simulink model "SS_F16_Block"  (Simulink 10.0)
settings: Solver=ode5  StartTime=0.0  StopTime=50  FixedStep=0.001  RelTol=1e-3  EnableMultiTasking=on
values from neighbouring files (symbols this model uses):
  A = A_lo    [augumentedF16.m]    (also in my_runLINF16sim.m; runLINF16sim.m)
  B = B_lo    [augumentedF16.m]    (also in my_runLINF16sim.m; runLINF16sim.m)
  C = C_lo    [augumentedF16.m]    (also in my_runLINF16sim.m; runLINF16sim.m)
  D = D_lo    [augumentedF16.m]    (also in my_runLINF16sim.m; runLINF16sim.m)
  DisAil_1 = AileronDis    (= 0)    [augumentedF16.m]    (also in my_runF16Sim.m; my_runLINF16sim.m; runF16Sim.m; runLINF16sim.m)
  DisAil_2 = -2*AileronDis    (= 0)    [augumentedF16.m]    (also in my_runF16Sim.m; my_runLINF16sim.m; runF16Sim.m; runLINF16sim.m)
  DisAil_3 = AileronDis    (= 0)    [augumentedF16.m]    (also in my_runF16Sim.m; my_runLINF16sim.m; runF16Sim.m; runLINF16sim.m)
  DisEle_1 = ElevatorDis    (= 0)    [augumentedF16.m]    (also in my_runF16Sim.m; my_runLINF16sim.m; runF16Sim.m; runLINF16sim.m)
  DisEle_2 = -2*ElevatorDis    (= 0)    [augumentedF16.m]    (also in my_runF16Sim.m; my_runLINF16sim.m; runF16Sim.m; runLINF16sim.m)
  DisEle_3 = ElevatorDis    (= 0)    [augumentedF16.m]    (also in my_runF16Sim.m; my_runLINF16sim.m; runF16Sim.m; runLINF16sim.m)
  DisRud_1 = RudderDis    (= 0)    [augumentedF16.m]    (also in my_runF16Sim.m; my_runLINF16sim.m; runF16Sim.m; runLINF16sim.m)
  DisRud_2 = -2*RudderDis    (= 0)    [augumentedF16.m]    (also in my_runF16Sim.m; my_runLINF16sim.m; runF16Sim.m; runLINF16sim.m)
  DisRud_3 = RudderDis    (= 0)    [augumentedF16.m]    (also in my_runF16Sim.m; my_runLINF16sim.m; runF16Sim.m; runLINF16sim.m)
  K = lqr(A_hi, B_hi, Q, R)    [augumentedF16.m]
  thrust = 5000    [FindF16Dynamics.m]    (also in augumentedF16.m = 0; my_FindF16Dynamics.m; my_runF16Sim.m; my_runLINF16sim.m = 0)
  trim_control = trim_control_lo    [augumentedF16.m]    (also in my_runLINF16sim.m; my_trim_F16.m = [xu(2);xu(4);xu(5)]; runLINF16sim.m)
  trim_thrust = trim_thrust_lo    [augumentedF16.m]    (also in my_runLINF16sim.m; my_trim_F16.m = xu(13); runLINF16sim.m)
settings Model: Creator=russ1110  LastModifiedBy=asmialek  ExtModeAutoUpdateStatusClock=off
settings DataIOCC: LimitDataPoints=on  SignalLoggingName=sigsOut
settings OptimizationCC: BooleanDataType=off  LifeSpan=auto
settings DebuggingCC: SaveWithParameterizedLinksMsg=none  SignalResolutionControl=TryResolveAllWithWarning  MultiTaskDSMMsg=warning  MultiTaskCondExecSysMsg=none  SFUnexpectedBacktrackingDiag=error  SFNoUnconditionalDefaultTransitionDiag=error  SFExecutionAtInitializationDiag=warning
settings HardwareCC: TargetUnknown=on
settings ConfigComp: CovExternalEMLEnable=off

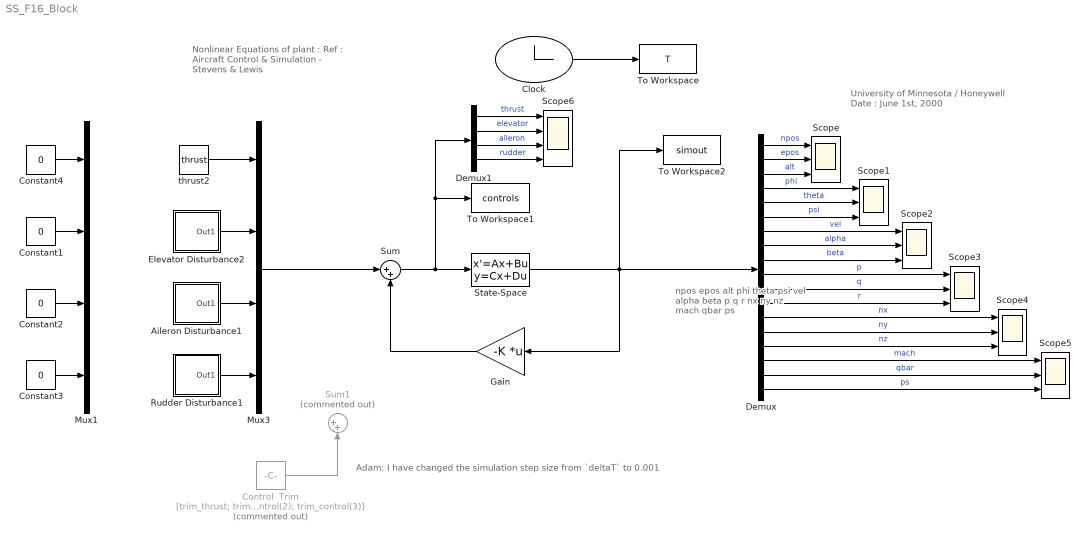
== system SS_F16_Block ==
  note: Adam: I have changed the simulation step size from `deltaT` to 0.001
  note: npos
      | epos
      | alt
      | phi
      | theta
      | psi
      | vel
      | alpha
      | beta
      | p
      | q
      | r
      | nx
      | ny
      | nz
      | mach
      | qbar
      | ps
  note: University of Minnesota / Honeywell
      | Date : June 1st, 2000
  note: Nonlinear Equations of plant :
      | Ref : Aircraft Control & Simulation
      | - Stevens & Lewis
  Aileron Disturbance1 : Subsystem
  Clock : Clock
      settings: Decimation=50
  Constant{1..4} (4 alike) : Constant  Value=0
  Control  Trim : Constant  Commented=on  Value=[trim_thrust; trim_control(1); trim_control(2); trim_control(3)]
  Demux : Demux  Outputs=18
  Demux1 : Demux
  Elevator Disturbance2 : Subsystem
  Gain : Gain  Gain=-K  Multiplication=Matrix(K*u)
  Mux1 : Mux
  Mux3 : Mux
  Rudder Disturbance1 : Subsystem
  Scope{,1..5} (6 alike) : Scope  NumInputPorts=3
  Scope6 : Scope  NumInputPorts=4
  State-Space : StateSpace  A=A  B=B  C=C  D=D  InitialCondition=0
  Sum : Sum  Inputs=|++
  Sum1 : Sum  Commented=on  Inputs=|++  SaturateOnIntegerOverflow=on  InputSameDT=on  OutDataTypeStr=Inherit: Same as first input
  To Workspace : ToWorkspace  VariableName=T  SampleTime=-1
      settings: Decimation=100
  To Workspace1 : ToWorkspace  VariableName=controls  SampleTime=-1
      settings: Decimation=100
  To Workspace2 : ToWorkspace  VariableName=simout  SampleTime=-1
      settings: Decimation=100
  thrust2 : Constant  Value=thrust  VectorParams1D=off
  wires:
  Clock/1 -> To Workspace/1
  Demux/1 -> Scope/1  "npos"
  Demux/2 -> Scope/2  "epos"
  Demux/3 -> Scope/3  "alt"
  Demux/5 -> Scope1/2  "theta"
  Demux/6 -> Scope1/3  "psi"
  Demux/7 -> Scope2/1  "vel"
  Demux/8 -> Scope2/2  "alpha"
  Demux/9 -> Scope2/3  "beta"
  Demux/10 -> Scope3/1  "p"
  Demux/11 -> Scope3/2  "q"
  Demux/12 -> Scope3/3  "r"
  Demux/13 -> Scope4/1  "nx"
  Demux/14 -> Scope4/2  "ny"
  Demux/15 -> Scope4/3  "nz"
  Demux/4 -> Scope1/1  "phi"
  Demux/16 -> Scope5/1  "mach"
  Demux/17 -> Scope5/2  "qbar"
  Demux/18 -> Scope5/3  "ps"
  Control  Trim/1 -> Sum1/2
  Constant1/1 -> Mux1/2
  Constant2/1 -> Mux1/3
  Constant3/1 -> Mux1/4
  Constant4/1 -> Mux1/1
  Demux1/4 -> Scope6/4  "rudder"
  Demux1/3 -> Scope6/3  "aileron"
  Demux1/2 -> Scope6/2  "elevator"
  Demux1/1 -> Scope6/1  "thrust"
  Sum/1 -> Demux1/1, To Workspace1/1, State-Space/1
  Gain/1 -> Sum/2
  State-Space/1 -> Gain/1, To Workspace2/1, Demux/1
  Elevator Disturbance2/1(Out1) -> Mux3/2
  thrust2/1 -> Mux3/1
  Rudder Disturbance1/1(Out1) -> Mux3/4
  Aileron Disturbance1/1(Out1) -> Mux3/3
  Mux3/1 -> Sum/1

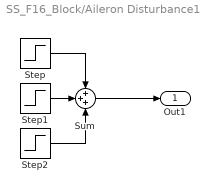
== system SS_F16_Block/Aileron Disturbance1 ==
  Step : Step  After=DisAil_1  SampleTime=0
  Step1 : Step  Time=3  After=DisAil_2  SampleTime=0
  Step2 : Step  Time=5  After=DisAil_3  SampleTime=0
  Sum : Sum  Inputs=+++  SaturateOnIntegerOverflow=on  InputSameDT=on  OutDataTypeStr=Inherit: Same as first input
  Out1 : Outport
  wires:
  Step1/1 -> Sum/2
  Step/1 -> Sum/1
  Step2/1 -> Sum/3
  Sum/1 -> Out1/1

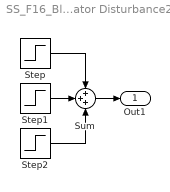
== system SS_F16_Block/Elevator Disturbance2 ==
  Step : Step  After=DisEle_1  SampleTime=0
  Step1 : Step  Time=3  After=DisEle_2  SampleTime=0
  Step2 : Step  Time=5  After=DisEle_3  SampleTime=0
  Sum : Sum  Inputs=+++  SaturateOnIntegerOverflow=on  InputSameDT=on  OutDataTypeStr=Inherit: Same as first input
  Out1 : Outport
  wires:
  Step1/1 -> Sum/2
  Step/1 -> Sum/1
  Step2/1 -> Sum/3
  Sum/1 -> Out1/1

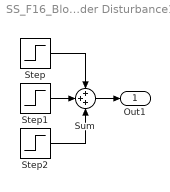
== system SS_F16_Block/Rudder Disturbance1 ==
  Step : Step  After=DisRud_1  SampleTime=0
  Step1 : Step  Time=1.5  After=DisRud_2  SampleTime=0
  Step2 : Step  Time=2  After=DisRud_3  SampleTime=0
  Sum : Sum  Inputs=+++  SaturateOnIntegerOverflow=on  InputSameDT=on  OutDataTypeStr=Inherit: Same as first input
  Out1 : Outport
  wires:
  Step1/1 -> Sum/2
  Step/1 -> Sum/1
  Step2/1 -> Sum/3
  Sum/1 -> Out1/1
